simulink model "sevietta_devel_2018a"  (R2013a)
settings: Solver=VariableStepDiscrete  SolverMode=SingleTasking  StartTime=0.0  StopTime=3276  RelTol=1e-3
undefined symbols (not defined in the file): sfp
libraries: xbsIndex_r4 x2589, casper_library_delays x40, simulink x19, casper_library_misc x17, xps_library x13
(part 17 of 32)

== system sevietta_devel_2018a/pkt/gbe3_start_chan ==
  sim_1 : Inport
  io_delay : xbsIndex_r4/Delay  rst=off  infoeditControl=Selection of Reset will increase slice count due to use of real FFs and instead of SRLs  en=off  latency=0  dbl_ovrd=off  reg_retiming=on  block_type=delay
  reint1 : xbsIndex_r4/Reinterpret  force_arith_type=on  arith_type=Unsigned  force_bin_pt=on  bin_pt=0  block_type=reinterpret
  sevietta_devel_2017k_pkt_gbe3_start_chan_user_data_out : xbsIndex_r4/Gateway In  gui_display_data_type=Fixed-point  arith_type=Unsigned  n_bits=32  bin_pt=0  preci_type=Single  exp_width=8  frac_width=24  quantization="Round  (unbiased: +/- Inf)"  overflow=Saturate  period=1  dbl_ovrd=off  timing_constraint=None  locs_specified=off  LOCs={}  UseAsADC=off  ADCChannel='1'  inherit_from_input=off  hdl_port=on  block_type=gatewayin
  slice_reg : xbsIndex_r4/Slice  nbits=16  boolean_output=off  mode=Lower Bit Location + Width  bit1=0  base1=MSB of Input  bit0=0  base0=LSB of Input  dbl_ovrd=off  block_type=slice
  in_reg : Outport
  wires:
  sevietta_devel_2017k_pkt_gbe3_start_chan_user_data_out/1 -> io_delay/1
  sim_1/1 -> sevietta_devel_2017k_pkt_gbe3_start_chan_user_data_out/1
  io_delay/1 -> slice_reg/1
  slice_reg/1 -> reint1/1
  reint1/1 -> in_reg/1

== system sevietta_devel_2018a/pkt/gbe3_stop_chan ==
  sim_1 : Inport
  io_delay : xbsIndex_r4/Delay  rst=off  infoeditControl=Selection of Reset will increase slice count due to use of real FFs and instead of SRLs  en=off  latency=0  dbl_ovrd=off  reg_retiming=on  block_type=delay
  reint1 : xbsIndex_r4/Reinterpret  force_arith_type=on  arith_type=Unsigned  force_bin_pt=on  bin_pt=0  block_type=reinterpret
  sevietta_devel_2017k_pkt_gbe3_stop_chan_user_data_out : xbsIndex_r4/Gateway In  gui_display_data_type=Fixed-point  arith_type=Unsigned  n_bits=32  bin_pt=0  preci_type=Single  exp_width=8  frac_width=24  quantization="Round  (unbiased: +/- Inf)"  overflow=Saturate  period=1  dbl_ovrd=off  timing_constraint=None  locs_specified=off  LOCs={}  UseAsADC=off  ADCChannel='1'  inherit_from_input=off  hdl_port=on  block_type=gatewayin
  slice_reg : xbsIndex_r4/Slice  nbits=16  boolean_output=off  mode=Lower Bit Location + Width  bit1=0  base1=MSB of Input  bit0=0  base0=LSB of Input  dbl_ovrd=off  block_type=slice
  in_reg : Outport
  wires:
  sevietta_devel_2017k_pkt_gbe3_stop_chan_user_data_out/1 -> io_delay/1
  sim_1/1 -> sevietta_devel_2017k_pkt_gbe3_stop_chan_user_data_out/1
  io_delay/1 -> slice_reg/1
  slice_reg/1 -> reint1/1
  reint1/1 -> in_reg/1

== system sevietta_devel_2018a/pkt/n_roach ==
  sim_1 : Inport
  io_delay : xbsIndex_r4/Delay  rst=off  infoeditControl=Selection of Reset will increase slice count due to use of real FFs and instead of SRLs  en=off  latency=0  dbl_ovrd=off  reg_retiming=on  block_type=delay
  reint1 : xbsIndex_r4/Reinterpret  force_arith_type=on  arith_type=Unsigned  force_bin_pt=on  bin_pt=0  block_type=reinterpret
  sevietta_devel_2017k_pkt_n_roach_user_data_out : xbsIndex_r4/Gateway In  gui_display_data_type=Fixed-point  arith_type=Unsigned  n_bits=32  bin_pt=0  preci_type=Single  exp_width=8  frac_width=24  quantization="Round  (unbiased: +/- Inf)"  overflow=Saturate  period=1  dbl_ovrd=off  timing_constraint=None  locs_specified=off  LOCs={}  UseAsADC=off  ADCChannel='1'  inherit_from_input=off  hdl_port=on  block_type=gatewayin
  slice_reg : xbsIndex_r4/Slice  nbits=32  boolean_output=off  mode=Lower Bit Location + Width  bit1=0  base1=MSB of Input  bit0=0  base0=LSB of Input  dbl_ovrd=off  block_type=slice
  in_reg : Outport
  wires:
  sevietta_devel_2017k_pkt_n_roach_user_data_out/1 -> io_delay/1
  sim_1/1 -> sevietta_devel_2017k_pkt_n_roach_user_data_out/1
  io_delay/1 -> slice_reg/1
  slice_reg/1 -> reint1/1
  reint1/1 -> in_reg/1

== system sevietta_devel_2018a/pkt/packetizer1 ==
  note: first channel ID is computed by re_logic for header
  note: do not go valid until after first FFT!
  note: Read enable for subband
      | extended by factor of 4 for
      | 256 -> 64 bit conversion
  note: all valid channels go into packet buffer
  note: make sure RE happens at start of window
  roach_id : Inport
  rst : Inport  Port=2
  new_fft_win : Inport  Port=3
  n_chanps : Inport  Port=4
  n_subband : Inport  Port=5
  data_in : Inport  Port=6
  data_valid : Inport  Port=7
  gbe_id : Inport  Port=8
  header_spare : Inport  Port=9
  first_chan : Inport  Port=10
  Delay{1,4..10} (8 alike) : xbsIndex_r4/Delay  rst=off  infoeditControl=Selection of Reset will increase slice count due to use of real FFs and instead of SRLs  en=off  latency=1  dbl_ovrd=off  reg_retiming=off  block_type=delay
  Delay3 : xbsIndex_r4/Delay  rst=off  infoeditControl=Selection of Reset will increase slice count due to use of real FFs and instead of SRLs  en=off  latency=8  dbl_ovrd=off  reg_retiming=off  block_type=delay
  Gateway Out{1..3,8,12} (5 alike) : xbsIndex_r4/Gateway Out  inherit_from_input=off  hdl_port=on  timing_constraint=None  locs_specified=off  LOCs={}  UseAsDAC=off  DACChannel='1'  block_type=gatewayout
  Inverter : xbsIndex_r4/Inverter  en=off  latency=0  dbl_ovrd=off  block_type=inv
  Logical : xbsIndex_r4/Logical  logical_function=OR  inputs=2  en=off  latency=0  precision=Full  arith_type=Unsigned  n_bits=16  bin_pt=0  align_bp=on  dbl_ovrd=off  block_type=logical
  Mux : xbsIndex_r4/Mux  inputs=2  en=off  latency=1  precision=Full  arith_type=Unsigned  n_bits=16  bin_pt=14  quantization=Truncate  overflow=Wrap  dbl_ovrd=off  block_type=mux
  Scope2 : Scope  NumInputPorts=5
      settings: ShowLegends=on  TimeRange=21.43365268244088  YMin=-5~0~-5~-5~-5  YMax=5~10~5~5~10  SaveName=ScopeData3  MaxDataPoints=10000
  n_chanps1 : InportShadow  Port=4
  n_subband1 : InportShadow  Port=5
  pkt_buffer : Subsystem
  pkt_header : Subsystem
  re_logic : Subsystem
  sync_delay : casper_library_delays/sync_delay  DelayLen=4096
  sync_delay1 : casper_library_delays/sync_delay  DelayLen=4096
  tx_data : Outport
  tx_valid : Outport  Port=2
  tx_eof : Outport  Port=3
  ip_addr_sel : Outport  Port=4
  wires:
  re_logic/6(pkt_chan0) -> [first_chan]
  header_spare/1 -> pkt_header/10(spare)
  [first_chan] -> pkt_header/9(first_chan)
  [subband_id] -> pkt_header/8(subband_id)
  re_logic/2(sub_id_out) -> ip_addr_sel/1, [subband_id]
  roach_id/1 -> pkt_header/4(roach_id)
  pkt_header/1(hdr_valid) -> Delay10/1, Delay9/1
  Delay1/1 -> Gateway Out3/1, tx_valid/1
  [pkt_eof] -> Delay3/1
  Gateway Out12/1 -> Scope2/5  "hdr data"
  re_logic/1(new_cycle_out) -> pkt_header/2(new_seq)
  re_logic/4(sof) -> pkt_header/3(new_pkt)
  pkt_header/2(hdr_out) -> Delay8/1
  Mux/1 -> Gateway Out2/1, tx_data/1
  Inverter/1 -> Gateway Out1/1, Mux/1
  Gateway Out1/1 -> Scope2/1  "hdr_buf_mux"
  Gateway Out2/1 -> Scope2/2  "data"
  Gateway Out3/1 -> Scope2/3  "pkt_valid"
  Gateway Out8/1 -> Scope2/4  "eof"
  Logical/1 -> Delay1/1, [pkt_valid]
  Delay3/1 -> Delay5/1
  gbe_id/1 -> pkt_header/5(gbe_id)
  n_chanps1/1 -> pkt_header/6(n_chan)
  n_subband1/1 -> pkt_header/7(n_subband)
  data_in/1 -> pkt_buffer/2(d_in)
  Delay9/1 -> Logical/1
  first_chan/1 -> re_logic/5(start_chan)
  rst/1 -> [rst], sync_delay1/1
  n_subband/1 -> re_logic/3(n_subband)
  n_chanps/1 -> re_logic/2(n_chanps)
  re_logic/5(eof) -> [pkt_eof]
  pkt_buffer/1(d_valid) -> Delay7/1
  pkt_buffer/2(d_out) -> Delay4/1
  Delay5/1 -> Delay6/1
  Delay6/1 -> Gateway Out8/1, tx_eof/1
  Delay4/1 -> Mux/3
  Delay7/1 -> Logical/2
  Delay8/1 -> Gateway Out12/1, Mux/2
  Delay10/1 -> Inverter/1
  new_fft_win/1 -> [new_fft_win], sync_delay/1
  [new_fft_win] -> pkt_buffer/4(new_fft_win)
  re_logic/3(sub_re) -> pkt_buffer/1(re)
  data_valid/1 -> pkt_buffer/3(we)
  [rst] -> pkt_header/1(rst)
  sync_delay/1 -> re_logic/1(sow)
  sync_delay1/1 -> re_logic/4(cnt_rst)

== system sevietta_devel_2018a/pkt/packetizer2 ==
  note: make sure RE happens at start of window
  note: all valid channels go into packet buffer
  note: Read enable for subband
      | extended by factor of 4 for
      | 256 -> 64 bit conversion
  note: do not go valid until after first FFT!
  note: first channel ID is computed by re_logic for header
  roach_id : Inport
  rst : Inport  Port=2
  new_fft_win : Inport  Port=3
  n_chanps : Inport  Port=4
  n_subband : Inport  Port=5
  data_in : Inport  Port=6
  data_valid : Inport  Port=7
  gbe_id : Inport  Port=8
  header_spare : Inport  Port=9
  first_chan : Inport  Port=10
  Delay{1,4..10} (8 alike) : xbsIndex_r4/Delay  rst=off  infoeditControl=Selection of Reset will increase slice count due to use of real FFs and instead of SRLs  en=off  latency=1  dbl_ovrd=off  reg_retiming=off  block_type=delay
  Delay3 : xbsIndex_r4/Delay  rst=off  infoeditControl=Selection of Reset will increase slice count due to use of real FFs and instead of SRLs  en=off  latency=8  dbl_ovrd=off  reg_retiming=off  block_type=delay
  Gateway Out{1..3,8,12} (5 alike) : xbsIndex_r4/Gateway Out  inherit_from_input=off  hdl_port=on  timing_constraint=None  locs_specified=off  LOCs={}  UseAsDAC=off  DACChannel='1'  block_type=gatewayout
  Inverter : xbsIndex_r4/Inverter  en=off  latency=0  dbl_ovrd=off  block_type=inv
  Logical : xbsIndex_r4/Logical  logical_function=OR  inputs=2  en=off  latency=0  precision=Full  arith_type=Unsigned  n_bits=16  bin_pt=0  align_bp=on  dbl_ovrd=off  block_type=logical
  Mux : xbsIndex_r4/Mux  inputs=2  en=off  latency=1  precision=Full  arith_type=Unsigned  n_bits=16  bin_pt=14  quantization=Truncate  overflow=Wrap  dbl_ovrd=off  block_type=mux
  Scope2 : Scope  NumInputPorts=5
      settings: ShowLegends=on  TimeRange=21.43365268244088  YMin=-5~0~-5~-5~-5  YMax=5~10~5~5~10  SaveName=ScopeData3  MaxDataPoints=10000
  n_chanps1 : InportShadow  Port=4
  n_subband1 : InportShadow  Port=5
  pkt_buffer : Subsystem
  pkt_header : Subsystem
  re_logic : Subsystem
  sync_delay : casper_library_delays/sync_delay  DelayLen=4096
  sync_delay1 : casper_library_delays/sync_delay  DelayLen=4096
  tx_data : Outport
  tx_valid : Outport  Port=2
  tx_eof : Outport  Port=3
  ip_addr_sel : Outport  Port=4
  wires:
  sync_delay1/1 -> re_logic/4(cnt_rst)
  sync_delay/1 -> re_logic/1(sow)
  [rst] -> pkt_header/1(rst)
  data_valid/1 -> pkt_buffer/3(we)
  re_logic/3(sub_re) -> pkt_buffer/1(re)
  [new_fft_win] -> pkt_buffer/4(new_fft_win)
  new_fft_win/1 -> sync_delay/1, [new_fft_win]
  Delay10/1 -> Inverter/1
  Delay8/1 -> Mux/2, Gateway Out12/1
  Delay7/1 -> Logical/2
  Delay4/1 -> Mux/3
  Delay6/1 -> tx_eof/1, Gateway Out8/1
  Delay5/1 -> Delay6/1
  pkt_buffer/2(d_out) -> Delay4/1
  pkt_buffer/1(d_valid) -> Delay7/1
  re_logic/5(eof) -> [pkt_eof]
  n_chanps/1 -> re_logic/2(n_chanps)
  n_subband/1 -> re_logic/3(n_subband)
  rst/1 -> sync_delay1/1, [rst]
  first_chan/1 -> re_logic/5(start_chan)
  Delay9/1 -> Logical/1
  data_in/1 -> pkt_buffer/2(d_in)
  n_subband1/1 -> pkt_header/7(n_subband)
  n_chanps1/1 -> pkt_header/6(n_chan)
  gbe_id/1 -> pkt_header/5(gbe_id)
  Delay3/1 -> Delay5/1
  Logical/1 -> [pkt_valid], Delay1/1
  Gateway Out8/1 -> Scope2/4  "eof"
  Gateway Out3/1 -> Scope2/3  "pkt_valid"
  Gateway Out2/1 -> Scope2/2  "data"
  Gateway Out1/1 -> Scope2/1  "hdr_buf_mux"
  Inverter/1 -> Mux/1, Gateway Out1/1
  Mux/1 -> tx_data/1, Gateway Out2/1
  pkt_header/2(hdr_out) -> Delay8/1
  re_logic/4(sof) -> pkt_header/3(new_pkt)
  re_logic/1(new_cycle_out) -> pkt_header/2(new_seq)
  Gateway Out12/1 -> Scope2/5  "hdr data"
  [pkt_eof] -> Delay3/1
  Delay1/1 -> tx_valid/1, Gateway Out3/1
  pkt_header/1(hdr_valid) -> Delay9/1, Delay10/1
  roach_id/1 -> pkt_header/4(roach_id)
  re_logic/2(sub_id_out) -> [subband_id], ip_addr_sel/1
  [subband_id] -> pkt_header/8(subband_id)
  [first_chan] -> pkt_header/9(first_chan)
  header_spare/1 -> pkt_header/10(spare)
  re_logic/6(pkt_chan0) -> [first_chan]

== system sevietta_devel_2018a/pkt/packetizer3 ==
  note: first channel ID is computed by re_logic for header
  note: do not go valid until after first FFT!
  note: Read enable for subband
      | extended by factor of 4 for
      | 256 -> 64 bit conversion
  note: all valid channels go into packet buffer
  note: make sure RE happens at start of window
  roach_id : Inport
  rst : Inport  Port=2
  new_fft_win : Inport  Port=3
  n_chanps : Inport  Port=4
  n_subband : Inport  Port=5
  data_in : Inport  Port=6
  data_valid : Inport  Port=7
  gbe_id : Inport  Port=8
  header_spare : Inport  Port=9
  first_chan : Inport  Port=10
  Delay{1,4..10} (8 alike) : xbsIndex_r4/Delay  rst=off  infoeditControl=Selection of Reset will increase slice count due to use of real FFs and instead of SRLs  en=off  latency=1  dbl_ovrd=off  reg_retiming=off  block_type=delay
  Delay3 : xbsIndex_r4/Delay  rst=off  infoeditControl=Selection of Reset will increase slice count due to use of real FFs and instead of SRLs  en=off  latency=8  dbl_ovrd=off  reg_retiming=off  block_type=delay
  Gateway Out{1..3,8,12} (5 alike) : xbsIndex_r4/Gateway Out  inherit_from_input=off  hdl_port=on  timing_constraint=None  locs_specified=off  LOCs={}  UseAsDAC=off  DACChannel='1'  block_type=gatewayout
  Inverter : xbsIndex_r4/Inverter  en=off  latency=0  dbl_ovrd=off  block_type=inv
  Logical : xbsIndex_r4/Logical  logical_function=OR  inputs=2  en=off  latency=0  precision=Full  arith_type=Unsigned  n_bits=16  bin_pt=0  align_bp=on  dbl_ovrd=off  block_type=logical
  Mux : xbsIndex_r4/Mux  inputs=2  en=off  latency=1  precision=Full  arith_type=Unsigned  n_bits=16  bin_pt=14  quantization=Truncate  overflow=Wrap  dbl_ovrd=off  block_type=mux
  Scope2 : Scope  NumInputPorts=5
      settings: ShowLegends=on  TimeRange=21.43365268244088  YMin=-5~0~-5~-5~-5  YMax=5~10~5~5~10  SaveName=ScopeData3  MaxDataPoints=10000
  n_chanps1 : InportShadow  Port=4
  n_subband1 : InportShadow  Port=5
  pkt_buffer : Subsystem
  pkt_header : Subsystem
  re_logic : Subsystem
  sync_delay : casper_library_delays/sync_delay  DelayLen=4096
  sync_delay1 : casper_library_delays/sync_delay  DelayLen=4096
  tx_data : Outport
  tx_valid : Outport  Port=2
  tx_eof : Outport  Port=3
  ip_addr_sel : Outport  Port=4
  wires:
  re_logic/6(pkt_chan0) -> [first_chan]
  header_spare/1 -> pkt_header/10(spare)
  [first_chan] -> pkt_header/9(first_chan)
  [subband_id] -> pkt_header/8(subband_id)
  re_logic/2(sub_id_out) -> ip_addr_sel/1, [subband_id]
  roach_id/1 -> pkt_header/4(roach_id)
  pkt_header/1(hdr_valid) -> Delay10/1, Delay9/1
  Delay1/1 -> Gateway Out3/1, tx_valid/1
  [pkt_eof] -> Delay3/1
  Gateway Out12/1 -> Scope2/5  "hdr data"
  re_logic/1(new_cycle_out) -> pkt_header/2(new_seq)
  re_logic/4(sof) -> pkt_header/3(new_pkt)
  pkt_header/2(hdr_out) -> Delay8/1
  Mux/1 -> Gateway Out2/1, tx_data/1
  Inverter/1 -> Gateway Out1/1, Mux/1
  Gateway Out1/1 -> Scope2/1  "hdr_buf_mux"
  Gateway Out2/1 -> Scope2/2  "data"
  Gateway Out3/1 -> Scope2/3  "pkt_valid"
  Gateway Out8/1 -> Scope2/4  "eof"
  Logical/1 -> Delay1/1, [pkt_valid]
  Delay3/1 -> Delay5/1
  gbe_id/1 -> pkt_header/5(gbe_id)
  n_chanps1/1 -> pkt_header/6(n_chan)
  n_subband1/1 -> pkt_header/7(n_subband)
  data_in/1 -> pkt_buffer/2(d_in)
  Delay9/1 -> Logical/1
  first_chan/1 -> re_logic/5(start_chan)
  rst/1 -> [rst], sync_delay1/1
  n_subband/1 -> re_logic/3(n_subband)
  n_chanps/1 -> re_logic/2(n_chanps)
  re_logic/5(eof) -> [pkt_eof]
  pkt_buffer/1(d_valid) -> Delay7/1
  pkt_buffer/2(d_out) -> Delay4/1
  Delay5/1 -> Delay6/1
  Delay6/1 -> Gateway Out8/1, tx_eof/1
  Delay4/1 -> Mux/3
  Delay7/1 -> Logical/2
  Delay8/1 -> Gateway Out12/1, Mux/2
  Delay10/1 -> Inverter/1
  new_fft_win/1 -> [new_fft_win], sync_delay/1
  [new_fft_win] -> pkt_buffer/4(new_fft_win)
  re_logic/3(sub_re) -> pkt_buffer/1(re)
  data_valid/1 -> pkt_buffer/3(we)
  [rst] -> pkt_header/1(rst)
  sync_delay/1 -> re_logic/1(sow)
  sync_delay1/1 -> re_logic/4(cnt_rst)

== system sevietta_devel_2018a/pkt/packetizer4 ==
  note: make sure RE happens at start of window
  note: all valid channels go into packet buffer
  note: Read enable for subband
      | extended by factor of 4 for
      | 256 -> 64 bit conversion
  note: do not go valid until after first FFT!
  note: first channel ID is computed by re_logic for header
  roach_id : Inport
  rst : Inport  Port=2
  new_fft_win : Inport  Port=3
  n_chanps : Inport  Port=4
  n_subband : Inport  Port=5
  data_in : Inport  Port=6
  data_valid : Inport  Port=7
  gbe_id : Inport  Port=8
  header_spare : Inport  Port=9
  first_chan : Inport  Port=10
  Delay{1,4..10} (8 alike) : xbsIndex_r4/Delay  rst=off  infoeditControl=Selection of Reset will increase slice count due to use of real FFs and instead of SRLs  en=off  latency=1  dbl_ovrd=off  reg_retiming=off  block_type=delay
  Delay3 : xbsIndex_r4/Delay  rst=off  infoeditControl=Selection of Reset will increase slice count due to use of real FFs and instead of SRLs  en=off  latency=8  dbl_ovrd=off  reg_retiming=off  block_type=delay
  Gateway Out{1..3,8,12} (5 alike) : xbsIndex_r4/Gateway Out  inherit_from_input=off  hdl_port=on  timing_constraint=None  locs_specified=off  LOCs={}  UseAsDAC=off  DACChannel='1'  block_type=gatewayout
  Inverter : xbsIndex_r4/Inverter  en=off  latency=0  dbl_ovrd=off  block_type=inv
  Logical : xbsIndex_r4/Logical  logical_function=OR  inputs=2  en=off  latency=0  precision=Full  arith_type=Unsigned  n_bits=16  bin_pt=0  align_bp=on  dbl_ovrd=off  block_type=logical
  Mux : xbsIndex_r4/Mux  inputs=2  en=off  latency=1  precision=Full  arith_type=Unsigned  n_bits=16  bin_pt=14  quantization=Truncate  overflow=Wrap  dbl_ovrd=off  block_type=mux
  Scope2 : Scope  NumInputPorts=5
      settings: ShowLegends=on  TimeRange=21.43365268244088  YMin=-5~0~-5~-5~-5  YMax=5~10~5~5~10  SaveName=ScopeData3  MaxDataPoints=10000
  n_chanps1 : InportShadow  Port=4
  n_subband1 : InportShadow  Port=5
  pkt_buffer : Subsystem
  pkt_header : Subsystem
  re_logic : Subsystem
  sync_delay : casper_library_delays/sync_delay  DelayLen=4096
  sync_delay1 : casper_library_delays/sync_delay  DelayLen=4096
  tx_data : Outport
  tx_valid : Outport  Port=2
  tx_eof : Outport  Port=3
  ip_addr_sel : Outport  Port=4
  wires:
  sync_delay1/1 -> re_logic/4(cnt_rst)
  sync_delay/1 -> re_logic/1(sow)
  [rst] -> pkt_header/1(rst)
  data_valid/1 -> pkt_buffer/3(we)
  re_logic/3(sub_re) -> pkt_buffer/1(re)
  [new_fft_win] -> pkt_buffer/4(new_fft_win)
  new_fft_win/1 -> sync_delay/1, [new_fft_win]
  Delay10/1 -> Inverter/1
  Delay8/1 -> Mux/2, Gateway Out12/1
  Delay7/1 -> Logical/2
  Delay4/1 -> Mux/3
  Delay6/1 -> tx_eof/1, Gateway Out8/1
  Delay5/1 -> Delay6/1
  pkt_buffer/2(d_out) -> Delay4/1
  pkt_buffer/1(d_valid) -> Delay7/1
  re_logic/5(eof) -> [pkt_eof]
  n_chanps/1 -> re_logic/2(n_chanps)
  n_subband/1 -> re_logic/3(n_subband)
  rst/1 -> sync_delay1/1, [rst]
  first_chan/1 -> re_logic/5(start_chan)
  Delay9/1 -> Logical/1
  data_in/1 -> pkt_buffer/2(d_in)
  n_subband1/1 -> pkt_header/7(n_subband)
  n_chanps1/1 -> pkt_header/6(n_chan)
  gbe_id/1 -> pkt_header/5(gbe_id)
  Delay3/1 -> Delay5/1
  Logical/1 -> [pkt_valid], Delay1/1
  Gateway Out8/1 -> Scope2/4  "eof"
  Gateway Out3/1 -> Scope2/3  "pkt_valid"
  Gateway Out2/1 -> Scope2/2  "data"
  Gateway Out1/1 -> Scope2/1  "hdr_buf_mux"
  Inverter/1 -> Mux/1, Gateway Out1/1
  Mux/1 -> tx_data/1, Gateway Out2/1
  pkt_header/2(hdr_out) -> Delay8/1
  re_logic/4(sof) -> pkt_header/3(new_pkt)
  re_logic/1(new_cycle_out) -> pkt_header/2(new_seq)
  Gateway Out12/1 -> Scope2/5  "hdr data"
  [pkt_eof] -> Delay3/1
  Delay1/1 -> tx_valid/1, Gateway Out3/1
  pkt_header/1(hdr_valid) -> Delay9/1, Delay10/1
  roach_id/1 -> pkt_header/4(roach_id)
  re_logic/2(sub_id_out) -> [subband_id], ip_addr_sel/1
  [subband_id] -> pkt_header/8(subband_id)
  [first_chan] -> pkt_header/9(first_chan)
  header_spare/1 -> pkt_header/10(spare)
  re_logic/6(pkt_chan0) -> [first_chan]

== system sevietta_devel_2018a/pkt/pipeline1 ==
  d : Inport
  Register0 : xbsIndex_r4/Register  init=0  rst=off  en=off  dbl_ovrd=off  block_type=register
      settings: block_version=11.4
  q : Outport
  wires:
  d/1 -> Register0/1
  Register0/1 -> q/1

== system sevietta_devel_2018a/pkt/pipeline10 ==
  d : Inport
  Register0 : xbsIndex_r4/Register  init=0  rst=off  en=off  dbl_ovrd=off  block_type=register
      settings: block_version=11.4
  q : Outport
  wires:
  d/1 -> Register0/1
  Register0/1 -> q/1

== system sevietta_devel_2018a/pkt/pipeline11 ==
  d : Inport
  Register0 : xbsIndex_r4/Register  init=0  rst=off  en=off  dbl_ovrd=off  block_type=register
      settings: block_version=11.4
  q : Outport
  wires:
  d/1 -> Register0/1
  Register0/1 -> q/1

== system sevietta_devel_2018a/pkt/pipeline12 ==
  d : Inport
  Register0 : xbsIndex_r4/Register  init=0  rst=off  en=off  dbl_ovrd=off  block_type=register
      settings: block_version=11.4
  q : Outport
  wires:
  d/1 -> Register0/1
  Register0/1 -> q/1

== system sevietta_devel_2018a/pkt/pipeline13 ==
  d : Inport
  Register0 : xbsIndex_r4/Register  init=0  rst=off  en=off  dbl_ovrd=off  block_type=register
      settings: block_version=11.4
  q : Outport
  wires:
  d/1 -> Register0/1
  Register0/1 -> q/1

== system sevietta_devel_2018a/pkt/pipeline14 ==
  d : Inport
  Register0 : xbsIndex_r4/Register  init=0  rst=off  en=off  dbl_ovrd=off  block_type=register
      settings: block_version=11.4
  q : Outport
  wires:
  d/1 -> Register0/1
  Register0/1 -> q/1

== system sevietta_devel_2018a/pkt/pipeline15 ==
  d : Inport
  Register0 : xbsIndex_r4/Register  init=0  rst=off  en=off  dbl_ovrd=off  block_type=register
      settings: block_version=11.4
  q : Outport
  wires:
  d/1 -> Register0/1
  Register0/1 -> q/1

== system sevietta_devel_2018a/pkt/pipeline16 ==
  d : Inport
  Register0 : xbsIndex_r4/Register  init=0  rst=off  en=off  dbl_ovrd=off  block_type=register
      settings: block_version=11.4
  q : Outport
  wires:
  d/1 -> Register0/1
  Register0/1 -> q/1

== system sevietta_devel_2018a/pkt/pipeline17 ==
  d : Inport
  Register0 : xbsIndex_r4/Register  init=0  rst=off  en=off  dbl_ovrd=off  block_type=register
      settings: block_version=11.4
  q : Outport
  wires:
  d/1 -> Register0/1
  Register0/1 -> q/1

== system sevietta_devel_2018a/pkt/pipeline18 ==
  d : Inport
  Register0 : xbsIndex_r4/Register  init=0  rst=off  en=off  dbl_ovrd=off  block_type=register
      settings: block_version=11.4
  q : Outport
  wires:
  d/1 -> Register0/1
  Register0/1 -> q/1

== system sevietta_devel_2018a/pkt/pipeline19 ==
  d : Inport
  Register0 : xbsIndex_r4/Register  init=0  rst=off  en=off  dbl_ovrd=off  block_type=register
      settings: block_version=11.4
  q : Outport
  wires:
  d/1 -> Register0/1
  Register0/1 -> q/1

== system sevietta_devel_2018a/pkt/pipeline2 ==
  d : Inport
  Register0 : xbsIndex_r4/Register  init=0  rst=off  en=off  dbl_ovrd=off  block_type=register
      settings: block_version=11.4
  q : Outport
  wires:
  d/1 -> Register0/1
  Register0/1 -> q/1

== system sevietta_devel_2018a/pkt/pipeline20 ==
  d : Inport
  Register0 : xbsIndex_r4/Register  init=0  rst=off  en=off  dbl_ovrd=off  block_type=register
      settings: block_version=11.4
  q : Outport
  wires:
  d/1 -> Register0/1
  Register0/1 -> q/1

== system sevietta_devel_2018a/pkt/pipeline21 ==
  d : Inport
  Register0 : xbsIndex_r4/Register  init=0  rst=off  en=off  dbl_ovrd=off  block_type=register
      settings: block_version=11.4
  q : Outport
  wires:
  d/1 -> Register0/1
  Register0/1 -> q/1

== system sevietta_devel_2018a/pkt/pipeline22 ==
  d : Inport
  Register0 : xbsIndex_r4/Register  init=0  rst=off  en=off  dbl_ovrd=off  block_type=register
      settings: block_version=11.4
  q : Outport
  wires:
  d/1 -> Register0/1
  Register0/1 -> q/1

== system sevietta_devel_2018a/pkt/pipeline23 ==
  d : Inport
  Register0 : xbsIndex_r4/Register  init=0  rst=off  en=off  dbl_ovrd=off  block_type=register
      settings: block_version=11.4
  q : Outport
  wires:
  d/1 -> Register0/1
  Register0/1 -> q/1

== system sevietta_devel_2018a/pkt/pipeline24 ==
  d : Inport
  Register0 : xbsIndex_r4/Register  init=0  rst=off  en=off  dbl_ovrd=off  block_type=register
      settings: block_version=11.4
  q : Outport
  wires:
  d/1 -> Register0/1
  Register0/1 -> q/1

== system sevietta_devel_2018a/pkt/pipeline25 ==
  d : Inport
  Register0 : xbsIndex_r4/Register  init=0  rst=off  en=off  dbl_ovrd=off  block_type=register
      settings: block_version=11.4
  q : Outport
  wires:
  d/1 -> Register0/1
  Register0/1 -> q/1

== system sevietta_devel_2018a/pkt/pipeline26 ==
  d : Inport
  Register0 : xbsIndex_r4/Register  init=0  rst=off  en=off  dbl_ovrd=off  block_type=register
      settings: block_version=11.4
  q : Outport
  wires:
  d/1 -> Register0/1
  Register0/1 -> q/1

== system sevietta_devel_2018a/pkt/pipeline27 ==
  d : Inport
  Register0 : xbsIndex_r4/Register  init=0  rst=off  en=off  dbl_ovrd=off  block_type=register
      settings: block_version=11.4
  q : Outport
  wires:
  d/1 -> Register0/1
  Register0/1 -> q/1

== system sevietta_devel_2018a/pkt/pipeline28 ==
  d : Inport
  Register0 : xbsIndex_r4/Register  init=0  rst=off  en=off  dbl_ovrd=off  block_type=register
      settings: block_version=11.4
  q : Outport
  wires:
  d/1 -> Register0/1
  Register0/1 -> q/1

== system sevietta_devel_2018a/pkt/pipeline29 ==
  d : Inport
  Register0 : xbsIndex_r4/Register  init=0  rst=off  en=off  dbl_ovrd=off  block_type=register
      settings: block_version=11.4
  q : Outport
  wires:
  d/1 -> Register0/1
  Register0/1 -> q/1

== system sevietta_devel_2018a/pkt/pipeline3 ==
  d : Inport
  Register0 : xbsIndex_r4/Register  init=0  rst=off  en=off  dbl_ovrd=off  block_type=register
      settings: block_version=11.4
  q : Outport
  wires:
  Register0/1 -> q/1
  d/1 -> Register0/1

== system sevietta_devel_2018a/pkt/pipeline30 ==
  d : Inport
  Register0 : xbsIndex_r4/Register  init=0  rst=off  en=off  dbl_ovrd=off  block_type=register
      settings: block_version=11.4
  q : Outport
  wires:
  d/1 -> Register0/1
  Register0/1 -> q/1

== system sevietta_devel_2018a/pkt/pipeline31 ==
  d : Inport
  Register0 : xbsIndex_r4/Register  init=0  rst=off  en=off  dbl_ovrd=off  block_type=register
      settings: block_version=11.4
  q : Outport
  wires:
  Register0/1 -> q/1
  d/1 -> Register0/1

== system sevietta_devel_2018a/pkt/pipeline32 ==
  d : Inport
  Register0 : xbsIndex_r4/Register  init=0  rst=off  en=off  dbl_ovrd=off  block_type=register
      settings: block_version=11.4
  q : Outport
  wires:
  d/1 -> Register0/1
  Register0/1 -> q/1

== system sevietta_devel_2018a/pkt/pipeline33 ==
  d : Inport
  Register0 : xbsIndex_r4/Register  init=0  rst=off  en=off  dbl_ovrd=off  block_type=register
      settings: block_version=11.4
  q : Outport
  wires:
  d/1 -> Register0/1
  Register0/1 -> q/1

== system sevietta_devel_2018a/pkt/pipeline34 ==
  d : Inport
  Register0 : xbsIndex_r4/Register  init=0  rst=off  en=off  dbl_ovrd=off  block_type=register
      settings: block_version=11.4
  q : Outport
  wires:
  d/1 -> Register0/1
  Register0/1 -> q/1

== system sevietta_devel_2018a/pkt/pipeline35 ==
  d : Inport
  Register0 : xbsIndex_r4/Register  init=0  rst=off  en=off  dbl_ovrd=off  block_type=register
      settings: block_version=11.4
  q : Outport
  wires:
  d/1 -> Register0/1
  Register0/1 -> q/1

== system sevietta_devel_2018a/pkt/pipeline36 ==
  d : Inport
  Register0 : xbsIndex_r4/Register  init=0  rst=off  en=off  dbl_ovrd=off  block_type=register
      settings: block_version=11.4
  q : Outport
  wires:
  d/1 -> Register0/1
  Register0/1 -> q/1

== system sevietta_devel_2018a/pkt/pipeline37 ==
  d : Inport
  Register0 : xbsIndex_r4/Register  init=0  rst=off  en=off  dbl_ovrd=off  block_type=register
      settings: block_version=11.4
  q : Outport
  wires:
  d/1 -> Register0/1
  Register0/1 -> q/1

== system sevietta_devel_2018a/pkt/pipeline38 ==
  d : Inport
  Register0 : xbsIndex_r4/Register  init=0  rst=off  en=off  dbl_ovrd=off  block_type=register
      settings: block_version=11.4
  q : Outport
  wires:
  d/1 -> Register0/1
  Register0/1 -> q/1

== system sevietta_devel_2018a/pkt/pipeline39 ==
  d : Inport
  Register0 : xbsIndex_r4/Register  init=0  rst=off  en=off  dbl_ovrd=off  block_type=register
      settings: block_version=11.4
  q : Outport
  wires:
  d/1 -> Register0/1
  Register0/1 -> q/1

== system sevietta_devel_2018a/pkt/pipeline4 ==
  d : Inport
  Register0 : xbsIndex_r4/Register  init=0  rst=off  en=off  dbl_ovrd=off  block_type=register
      settings: block_version=11.4
  q : Outport
  wires:
  d/1 -> Register0/1
  Register0/1 -> q/1

== system sevietta_devel_2018a/pkt/pipeline40 ==
  d : Inport
  Register0 : xbsIndex_r4/Register  init=0  rst=off  en=off  dbl_ovrd=off  block_type=register
      settings: block_version=11.4
  q : Outport
  wires:
  Register0/1 -> q/1
  d/1 -> Register0/1

== system sevietta_devel_2018a/pkt/pipeline41 ==
  d : Inport
  Register0 : xbsIndex_r4/Register  init=0  rst=off  en=off  dbl_ovrd=off  block_type=register
      settings: block_version=11.4
  q : Outport
  wires:
  d/1 -> Register0/1
  Register0/1 -> q/1

== system sevietta_devel_2018a/pkt/pipeline42 ==
  d : Inport
  Register0 : xbsIndex_r4/Register  init=0  rst=off  en=off  dbl_ovrd=off  block_type=register
      settings: block_version=11.4
  q : Outport
  wires:
  Register0/1 -> q/1
  d/1 -> Register0/1

== system sevietta_devel_2018a/pkt/pipeline43 ==
  d : Inport
  Register0 : xbsIndex_r4/Register  init=0  rst=off  en=off  dbl_ovrd=off  block_type=register
      settings: block_version=11.4
  q : Outport
  wires:
  d/1 -> Register0/1
  Register0/1 -> q/1

== system sevietta_devel_2018a/pkt/pipeline44 ==
  d : Inport
  Register0 : xbsIndex_r4/Register  init=0  rst=off  en=off  dbl_ovrd=off  block_type=register
      settings: block_version=11.4
  q : Outport
  wires:
  Register0/1 -> q/1
  d/1 -> Register0/1

== system sevietta_devel_2018a/pkt/pipeline45 ==
  d : Inport
  Register0 : xbsIndex_r4/Register  init=0  rst=off  en=off  dbl_ovrd=off  block_type=register
      settings: block_version=11.4
  q : Outport
  wires:
  d/1 -> Register0/1
  Register0/1 -> q/1

== system sevietta_devel_2018a/pkt/pipeline46 ==
  d : Inport
  Register0 : xbsIndex_r4/Register  init=0  rst=off  en=off  dbl_ovrd=off  block_type=register
      settings: block_version=11.4
  q : Outport
  wires:
  Register0/1 -> q/1
  d/1 -> Register0/1

== system sevietta_devel_2018a/pkt/pipeline47 ==
  d : Inport
  Register0 : xbsIndex_r4/Register  init=0  rst=off  en=off  dbl_ovrd=off  block_type=register
      settings: block_version=11.4
  q : Outport
  wires:
  Register0/1 -> q/1
  d/1 -> Register0/1

== system sevietta_devel_2018a/pkt/pipeline48 ==
  d : Inport
  Register0 : xbsIndex_r4/Register  init=0  rst=off  en=off  dbl_ovrd=off  block_type=register
      settings: block_version=11.4
  q : Outport
  wires:
  Register0/1 -> q/1
  d/1 -> Register0/1

== system sevietta_devel_2018a/pkt/pipeline49 ==
  d : Inport
  Register0 : xbsIndex_r4/Register  init=0  rst=off  en=off  dbl_ovrd=off  block_type=register
      settings: block_version=11.4
  q : Outport
  wires:
  Register0/1 -> q/1
  d/1 -> Register0/1

== system sevietta_devel_2018a/pkt/pipeline5 ==
  d : Inport
  Register0 : xbsIndex_r4/Register  init=0  rst=off  en=off  dbl_ovrd=off  block_type=register
      settings: block_version=11.4
  q : Outport
  wires:
  d/1 -> Register0/1
  Register0/1 -> q/1

== system sevietta_devel_2018a/pkt/pipeline50 ==
  d : Inport
  Register0 : xbsIndex_r4/Register  init=0  rst=off  en=off  dbl_ovrd=off  block_type=register
      settings: block_version=11.4
  q : Outport
  wires:
  Register0/1 -> q/1
  d/1 -> Register0/1

== system sevietta_devel_2018a/pkt/pipeline51 ==
  d : Inport
  Register0 : xbsIndex_r4/Register  init=0  rst=off  en=off  dbl_ovrd=off  block_type=register
      settings: block_version=11.4
  q : Outport
  wires:
  Register0/1 -> q/1
  d/1 -> Register0/1

== system sevietta_devel_2018a/pkt/pipeline52 ==
  d : Inport
  Register0 : xbsIndex_r4/Register  init=0  rst=off  en=off  dbl_ovrd=off  block_type=register
      settings: block_version=11.4
  q : Outport
  wires:
  Register0/1 -> q/1
  d/1 -> Register0/1

== system sevietta_devel_2018a/pkt/pipeline53 ==
  d : Inport
  Register0 : xbsIndex_r4/Register  init=0  rst=off  en=off  dbl_ovrd=off  block_type=register
      settings: block_version=11.4
  q : Outport
  wires:
  Register0/1 -> q/1
  d/1 -> Register0/1

== system sevietta_devel_2018a/pkt/pipeline54 ==
  d : Inport
  Register0 : xbsIndex_r4/Register  init=0  rst=off  en=off  dbl_ovrd=off  block_type=register
      settings: block_version=11.4
  q : Outport
  wires:
  Register0/1 -> q/1
  d/1 -> Register0/1

== system sevietta_devel_2018a/pkt/pipeline55 ==
  d : Inport
  Register0 : xbsIndex_r4/Register  init=0  rst=off  en=off  dbl_ovrd=off  block_type=register
      settings: block_version=11.4
  q : Outport
  wires:
  d/1 -> Register0/1
  Register0/1 -> q/1

== system sevietta_devel_2018a/pkt/pipeline56 ==
  d : Inport
  Register0 : xbsIndex_r4/Register  init=0  rst=off  en=off  dbl_ovrd=off  block_type=register
      settings: block_version=11.4
  q : Outport
  wires:
  Register0/1 -> q/1
  d/1 -> Register0/1

== system sevietta_devel_2018a/pkt/pipeline57 ==
  d : Inport
  Register0 : xbsIndex_r4/Register  init=0  rst=off  en=off  dbl_ovrd=off  block_type=register
      settings: block_version=11.4
  q : Outport
  wires:
  d/1 -> Register0/1
  Register0/1 -> q/1

== system sevietta_devel_2018a/pkt/pipeline58 ==
  d : Inport
  Register0 : xbsIndex_r4/Register  init=0  rst=off  en=off  dbl_ovrd=off  block_type=register
      settings: block_version=11.4
  q : Outport
  wires:
  Register0/1 -> q/1
  d/1 -> Register0/1

== system sevietta_devel_2018a/pkt/pipeline59 ==
  d : Inport
  Register0 : xbsIndex_r4/Register  init=0  rst=off  en=off  dbl_ovrd=off  block_type=register
      settings: block_version=11.4
  q : Outport
  wires:
  Register0/1 -> q/1
  d/1 -> Register0/1

== system sevietta_devel_2018a/pkt/pipeline6 ==
  d : Inport
  Register0 : xbsIndex_r4/Register  init=0  rst=off  en=off  dbl_ovrd=off  block_type=register
      settings: block_version=11.4
  q : Outport
  wires:
  d/1 -> Register0/1
  Register0/1 -> q/1

== system sevietta_devel_2018a/pkt/pipeline60 ==
  d : Inport
  Register0 : xbsIndex_r4/Register  init=0  rst=off  en=off  dbl_ovrd=off  block_type=register
      settings: block_version=11.4
  q : Outport
  wires:
  Register0/1 -> q/1
  d/1 -> Register0/1

== system sevietta_devel_2018a/pkt/pipeline61 ==
  d : Inport
  Register0 : xbsIndex_r4/Register  init=0  rst=off  en=off  dbl_ovrd=off  block_type=register
      settings: block_version=11.4
  q : Outport
  wires:
  Register0/1 -> q/1
  d/1 -> Register0/1

== system sevietta_devel_2018a/pkt/pipeline62 ==
  d : Inport
  Register0 : xbsIndex_r4/Register  init=0  rst=off  en=off  dbl_ovrd=off  block_type=register
      settings: block_version=11.4
  q : Outport
  wires:
  Register0/1 -> q/1
  d/1 -> Register0/1

== system sevietta_devel_2018a/pkt/pipeline63 ==
  d : Inport
  Register0 : xbsIndex_r4/Register  init=0  rst=off  en=off  dbl_ovrd=off  block_type=register
      settings: block_version=11.4
  q : Outport
  wires:
  Register0/1 -> q/1
  d/1 -> Register0/1

== system sevietta_devel_2018a/pkt/pipeline64 ==
  d : Inport
  Register0 : xbsIndex_r4/Register  init=0  rst=off  en=off  dbl_ovrd=off  block_type=register
      settings: block_version=11.4
  q : Outport
  wires:
  Register0/1 -> q/1
  d/1 -> Register0/1

== system sevietta_devel_2018a/pkt/pipeline65 ==
  d : Inport
  Register0 : xbsIndex_r4/Register  init=0  rst=off  en=off  dbl_ovrd=off  block_type=register
      settings: block_version=11.4
  q : Outport
  wires:
  d/1 -> Register0/1
  Register0/1 -> q/1

== system sevietta_devel_2018a/pkt/pipeline66 ==
  d : Inport
  Register0 : xbsIndex_r4/Register  init=0  rst=off  en=off  dbl_ovrd=off  block_type=register
      settings: block_version=11.4
  q : Outport
  wires:
  d/1 -> Register0/1
  Register0/1 -> q/1

== system sevietta_devel_2018a/pkt/pipeline67 ==
  d : Inport
  Register0 : xbsIndex_r4/Register  init=0  rst=off  en=off  dbl_ovrd=off  block_type=register
      settings: block_version=11.4
  q : Outport
  wires:
  d/1 -> Register0/1
  Register0/1 -> q/1

== system sevietta_devel_2018a/pkt/pipeline68 ==
  d : Inport
  Register0 : xbsIndex_r4/Register  init=0  rst=off  en=off  dbl_ovrd=off  block_type=register
      settings: block_version=11.4
  q : Outport
  wires:
  d/1 -> Register0/1
  Register0/1 -> q/1

== system sevietta_devel_2018a/pkt/pipeline69 ==
  d : Inport
  Register0 : xbsIndex_r4/Register  init=0  rst=off  en=off  dbl_ovrd=off  block_type=register
      settings: block_version=11.4
  q : Outport
  wires:
  d/1 -> Register0/1
  Register0/1 -> q/1

== system sevietta_devel_2018a/pkt/pipeline7 ==
  d : Inport
  Register0 : xbsIndex_r4/Register  init=0  rst=off  en=off  dbl_ovrd=off  block_type=register
      settings: block_version=11.4
  q : Outport
  wires:
  d/1 -> Register0/1
  Register0/1 -> q/1

== system sevietta_devel_2018a/pkt/pipeline70 ==
  d : Inport
  Register0 : xbsIndex_r4/Register  init=0  rst=off  en=off  dbl_ovrd=off  block_type=register
      settings: block_version=11.4
  q : Outport
  wires:
  d/1 -> Register0/1
  Register0/1 -> q/1

== system sevietta_devel_2018a/pkt/pipeline71 ==
  d : Inport
  Register0 : xbsIndex_r4/Register  init=0  rst=off  en=off  dbl_ovrd=off  block_type=register
      settings: block_version=11.4
  q : Outport
  wires:
  d/1 -> Register0/1
  Register0/1 -> q/1

== system sevietta_devel_2018a/pkt/pipeline72 ==
  d : Inport
  Register0 : xbsIndex_r4/Register  init=0  rst=off  en=off  dbl_ovrd=off  block_type=register
      settings: block_version=11.4
  q : Outport
  wires:
  d/1 -> Register0/1
  Register0/1 -> q/1

== system sevietta_devel_2018a/pkt/pipeline73 ==
  d : Inport
  Register0 : xbsIndex_r4/Register  init=0  rst=off  en=off  dbl_ovrd=off  block_type=register
      settings: block_version=11.4
  q : Outport
  wires:
  d/1 -> Register0/1
  Register0/1 -> q/1

== system sevietta_devel_2018a/pkt/pipeline74 ==
  d : Inport
  Register0 : xbsIndex_r4/Register  init=0  rst=off  en=off  dbl_ovrd=off  block_type=register
      settings: block_version=11.4
  q : Outport
  wires:
  Register0/1 -> q/1
  d/1 -> Register0/1

== system sevietta_devel_2018a/pkt/pipeline75 ==
  d : Inport
  Register0 : xbsIndex_r4/Register  init=0  rst=off  en=off  dbl_ovrd=off  block_type=register
      settings: block_version=11.4
  q : Outport
  wires:
  d/1 -> Register0/1
  Register0/1 -> q/1

== system sevietta_devel_2018a/pkt/pipeline76 ==
  d : Inport
  Register0 : xbsIndex_r4/Register  init=0  rst=off  en=off  dbl_ovrd=off  block_type=register
      settings: block_version=11.4
  q : Outport
  wires:
  Register0/1 -> q/1
  d/1 -> Register0/1

== system sevietta_devel_2018a/pkt/pipeline77 ==
  d : Inport
  Register0 : xbsIndex_r4/Register  init=0  rst=off  en=off  dbl_ovrd=off  block_type=register
      settings: block_version=11.4
  q : Outport
  wires:
  d/1 -> Register0/1
  Register0/1 -> q/1

== system sevietta_devel_2018a/pkt/pipeline78 ==
  d : Inport
  Register0 : xbsIndex_r4/Register  init=0  rst=off  en=off  dbl_ovrd=off  block_type=register
      settings: block_version=11.4
  q : Outport
  wires:
  d/1 -> Register0/1
  Register0/1 -> q/1

== system sevietta_devel_2018a/pkt/pipeline79 ==
  d : Inport
  Register0 : xbsIndex_r4/Register  init=0  rst=off  en=off  dbl_ovrd=off  block_type=register
      settings: block_version=11.4
  q : Outport
  wires:
  d/1 -> Register0/1
  Register0/1 -> q/1

== system sevietta_devel_2018a/pkt/pipeline8 ==
  d : Inport
  Register0 : xbsIndex_r4/Register  init=0  rst=off  en=off  dbl_ovrd=off  block_type=register
      settings: block_version=11.4
  q : Outport
  wires:
  d/1 -> Register0/1
  Register0/1 -> q/1

== system sevietta_devel_2018a/pkt/pipeline80 ==
  d : Inport
  Register0 : xbsIndex_r4/Register  init=0  rst=off  en=off  dbl_ovrd=off  block_type=register
      settings: block_version=11.4
  q : Outport
  wires:
  d/1 -> Register0/1
  Register0/1 -> q/1

== system sevietta_devel_2018a/pkt/pipeline81 ==
  d : Inport
  Register0 : xbsIndex_r4/Register  init=0  rst=off  en=off  dbl_ovrd=off  block_type=register
      settings: block_version=11.4
  q : Outport
  wires:
  d/1 -> Register0/1
  Register0/1 -> q/1

== system sevietta_devel_2018a/pkt/pipeline82 ==
  d : Inport
  Register0 : xbsIndex_r4/Register  init=0  rst=off  en=off  dbl_ovrd=off  block_type=register
      settings: block_version=11.4
  q : Outport
  wires:
  d/1 -> Register0/1
  Register0/1 -> q/1

== system sevietta_devel_2018a/pkt/pipeline83 ==
  d : Inport
  Register0 : xbsIndex_r4/Register  init=0  rst=off  en=off  dbl_ovrd=off  block_type=register
      settings: block_version=11.4
  q : Outport
  wires:
  d/1 -> Register0/1
  Register0/1 -> q/1

== system sevietta_devel_2018a/pkt/pipeline84 ==
  d : Inport
  Register0 : xbsIndex_r4/Register  init=0  rst=off  en=off  dbl_ovrd=off  block_type=register
      settings: block_version=11.4
  q : Outport
  wires:
  d/1 -> Register0/1
  Register0/1 -> q/1

== system sevietta_devel_2018a/pkt/pipeline9 ==
  d : Inport
  Register0 : xbsIndex_r4/Register  init=0  rst=off  en=off  dbl_ovrd=off  block_type=register
      settings: block_version=11.4
  q : Outport
  wires:
  d/1 -> Register0/1
  Register0/1 -> q/1

== system sevietta_devel_2018a/pkt/regup1 ==
  note: Invert so only goes high once, not every window
  sync_in : Inport
  d_in : Inport  Port=2
  Register : xbsIndex_r4/Register  init=0  rst=off  en=on  dbl_ovrd=off  block_type=register
  d_out : Outport
  wires:
  Register/1 -> d_out/1
  d_in/1 -> Register/1
  sync_in/1 -> Register/2

== system sevietta_devel_2018a/pkt/regup10 ==
  note: Invert so only goes high once, not every window
  sync_in : Inport
  d_in : Inport  Port=2
  Register : xbsIndex_r4/Register  init=0  rst=off  en=on  dbl_ovrd=off  block_type=register
  d_out : Outport
  wires:
  sync_in/1 -> Register/2
  d_in/1 -> Register/1
  Register/1 -> d_out/1

== system sevietta_devel_2018a/pkt/regup11 ==
  note: Invert so only goes high once, not every window
  sync_in : Inport
  d_in : Inport  Port=2
  Register : xbsIndex_r4/Register  init=0  rst=off  en=on  dbl_ovrd=off  block_type=register
  d_out : Outport
  wires:
  sync_in/1 -> Register/2
  d_in/1 -> Register/1
  Register/1 -> d_out/1

== system sevietta_devel_2018a/pkt/regup12 ==
  note: Invert so only goes high once, not every window
  sync_in : Inport
  d_in : Inport  Port=2
  Register : xbsIndex_r4/Register  init=0  rst=off  en=on  dbl_ovrd=off  block_type=register
  d_out : Outport
  wires:
  sync_in/1 -> Register/2
  d_in/1 -> Register/1
  Register/1 -> d_out/1

== system sevietta_devel_2018a/pkt/regup13 ==
  note: Invert so only goes high once, not every window
  sync_in : Inport
  d_in : Inport  Port=2
  Register : xbsIndex_r4/Register  init=0  rst=off  en=on  dbl_ovrd=off  block_type=register
  d_out : Outport
  wires:
  sync_in/1 -> Register/2
  d_in/1 -> Register/1
  Register/1 -> d_out/1

== system sevietta_devel_2018a/pkt/regup14 ==
  note: Invert so only goes high once, not every window
  sync_in : Inport
  d_in : Inport  Port=2
  Register : xbsIndex_r4/Register  init=0  rst=off  en=on  dbl_ovrd=off  block_type=register
  d_out : Outport
  wires:
  Register/1 -> d_out/1
  d_in/1 -> Register/1
  sync_in/1 -> Register/2

== system sevietta_devel_2018a/pkt/regup15 ==
  note: Invert so only goes high once, not every window
  sync_in : Inport
  d_in : Inport  Port=2
  Register : xbsIndex_r4/Register  init=0  rst=off  en=on  dbl_ovrd=off  block_type=register
  d_out : Outport
  wires:
  sync_in/1 -> Register/2
  d_in/1 -> Register/1
  Register/1 -> d_out/1

== system sevietta_devel_2018a/pkt/regup16 ==
  note: Invert so only goes high once, not every window
  sync_in : Inport
  d_in : Inport  Port=2
  Register : xbsIndex_r4/Register  init=0  rst=off  en=on  dbl_ovrd=off  block_type=register
  d_out : Outport
  wires:
  Register/1 -> d_out/1
  d_in/1 -> Register/1
  sync_in/1 -> Register/2

== system sevietta_devel_2018a/pkt/regup17 ==
  note: Invert so only goes high once, not every window
  sync_in : Inport
  d_in : Inport  Port=2
  Register : xbsIndex_r4/Register  init=0  rst=off  en=on  dbl_ovrd=off  block_type=register
  d_out : Outport
  wires:
  Register/1 -> d_out/1
  d_in/1 -> Register/1
  sync_in/1 -> Register/2

== system sevietta_devel_2018a/pkt/regup2 ==
  note: Invert so only goes high once, not every window
  sync_in : Inport
  d_in : Inport  Port=2
  Register : xbsIndex_r4/Register  init=0  rst=off  en=on  dbl_ovrd=off  block_type=register
  d_out : Outport
  wires:
  Register/1 -> d_out/1
  d_in/1 -> Register/1
  sync_in/1 -> Register/2

== system sevietta_devel_2018a/pkt/regup3 ==
  note: Invert so only goes high once, not every window
  sync_in : Inport
  d_in : Inport  Port=2
  Register : xbsIndex_r4/Register  init=0  rst=off  en=on  dbl_ovrd=off  block_type=register
  d_out : Outport
  wires:
  sync_in/1 -> Register/2
  d_in/1 -> Register/1
  Register/1 -> d_out/1

== system sevietta_devel_2018a/pkt/regup4 ==
  note: Invert so only goes high once, not every window
  sync_in : Inport
  d_in : Inport  Port=2
  Register : xbsIndex_r4/Register  init=0  rst=off  en=on  dbl_ovrd=off  block_type=register
  d_out : Outport
  wires:
  Register/1 -> d_out/1
  d_in/1 -> Register/1
  sync_in/1 -> Register/2

== system sevietta_devel_2018a/pkt/regup5 ==
  note: Invert so only goes high once, not every window
  sync_in : Inport
  d_in : Inport  Port=2
  Register : xbsIndex_r4/Register  init=0  rst=off  en=on  dbl_ovrd=off  block_type=register
  d_out : Outport
  wires:
  sync_in/1 -> Register/2
  d_in/1 -> Register/1
  Register/1 -> d_out/1

== system sevietta_devel_2018a/pkt/regup6 ==
  note: Invert so only goes high once, not every window
  sync_in : Inport
  d_in : Inport  Port=2
  Register : xbsIndex_r4/Register  init=0  rst=off  en=on  dbl_ovrd=off  block_type=register
  d_out : Outport
  wires:
  Register/1 -> d_out/1
  d_in/1 -> Register/1
  sync_in/1 -> Register/2

== system sevietta_devel_2018a/pkt/regup7 ==
  note: Invert so only goes high once, not every window
  sync_in : Inport
  d_in : Inport  Port=2
  Register : xbsIndex_r4/Register  init=0  rst=off  en=on  dbl_ovrd=off  block_type=register
  d_out : Outport
  wires:
  Register/1 -> d_out/1
  d_in/1 -> Register/1
  sync_in/1 -> Register/2

== system sevietta_devel_2018a/pkt/regup8 ==
  note: Invert so only goes high once, not every window
  sync_in : Inport
  d_in : Inport  Port=2
  Register : xbsIndex_r4/Register  init=0  rst=off  en=on  dbl_ovrd=off  block_type=register
  d_out : Outport
  wires:
  sync_in/1 -> Register/2
  d_in/1 -> Register/1
  Register/1 -> d_out/1

== system sevietta_devel_2018a/pkt/regup9 ==
  note: Invert so only goes high once, not every window
  sync_in : Inport
  d_in : Inport  Port=2
  Register : xbsIndex_r4/Register  init=0  rst=off  en=on  dbl_ovrd=off  block_type=register
  d_out : Outport
  wires:
  Register/1 -> d_out/1
  d_in/1 -> Register/1
  sync_in/1 -> Register/2

== system sevietta_devel_2018a/pkt/roach_id ==
  sim_1 : Inport
  io_delay : xbsIndex_r4/Delay  rst=off  infoeditControl=Selection of Reset will increase slice count due to use of real FFs and instead of SRLs  en=off  latency=0  dbl_ovrd=off  reg_retiming=on  block_type=delay
  reint1 : xbsIndex_r4/Reinterpret  force_arith_type=on  arith_type=Unsigned  force_bin_pt=on  bin_pt=0  block_type=reinterpret
  sevietta_devel_2017k_pkt_roach_id_user_data_out : xbsIndex_r4/Gateway In  gui_display_data_type=Fixed-point  arith_type=Unsigned  n_bits=32  bin_pt=0  preci_type=Single  exp_width=8  frac_width=24  quantization="Round  (unbiased: +/- Inf)"  overflow=Saturate  period=1  dbl_ovrd=off  timing_constraint=None  locs_specified=off  LOCs={}  UseAsADC=off  ADCChannel='1'  inherit_from_input=off  hdl_port=on  block_type=gatewayin
  slice_reg : xbsIndex_r4/Slice  nbits=32  boolean_output=off  mode=Lower Bit Location + Width  bit1=0  base1=MSB of Input  bit0=0  base0=LSB of Input  dbl_ovrd=off  block_type=slice
  in_reg : Outport
  wires:
  sevietta_devel_2017k_pkt_roach_id_user_data_out/1 -> io_delay/1
  sim_1/1 -> sevietta_devel_2017k_pkt_roach_id_user_data_out/1
  io_delay/1 -> slice_reg/1
  slice_reg/1 -> reint1/1
  reint1/1 -> in_reg/1
